simulink model "genset_imp_1"  (Simulink 7.6)
settings: Solver=ode23t  StartTime=0.0  StopTime=1  RelTol=1e-3
values from neighbouring files (symbols this model uses):
  AvrSat = 20*sqrt(2/3)    [articlerun.m]
  D_fw = 0.0    (= 0)    [articlerun.m]    (also in m1.m = 0.01)
  Davr = 0    [articlerun.m]
  Dgovernor = 10    [articlerun.m]
  droopAVR = 0.05    [articlerun.m]    (also in m1.m)
  droopGovernor = 0    [articlerun.m]    (also in m1.m)
  GovernorSamp = .01    (= 0.01)    [articlerun.m]
  H = 5.6    [articlerun.m]    (also in m1.m = 0.5*J_rotor*wbasem*wbasem/Sbase)
  Iavr = 0    [articlerun.m]
  Igovernor = 10    [articlerun.m]
  loadAmplitude = 0    [initArt.m]
  loadBias = 0.5    [initArt.m]
  loadfreq = 2*pi/loadT    (= 628.318530718)    [initArt.m]
  loadStep = 0    [initArt.m]
  loadStepTime = 15    [initArt.m]
  Pavr = 400    [articlerun.m]
  Pgovernor = 20    [articlerun.m]
  S_b = 325e6    (= 325000000)    [articlerun.m]    (also in m1.m)
  V_b = 26e3    (= 26000)    [articlerun.m]    (also in m1.m = 20000)
  w_b = 60*2*pi    (= 376.991118431)    [articlerun.m]    (also in m1.m)
undefined symbols (not defined in the file or in its folder): delayEngineRack, deltaomega, Genset, PMSlib, R_a, tau_e, Xbus
libraries: simulink x2
settings Model: Creator=tibnor  LastModifiedBy=tibnor  BufferReuse=off
settings OptimizationCC: OptimizeBlockIOStorage=off  BufferReuse=off  ExpressionFolding=off  LocalBlockOutputs=off

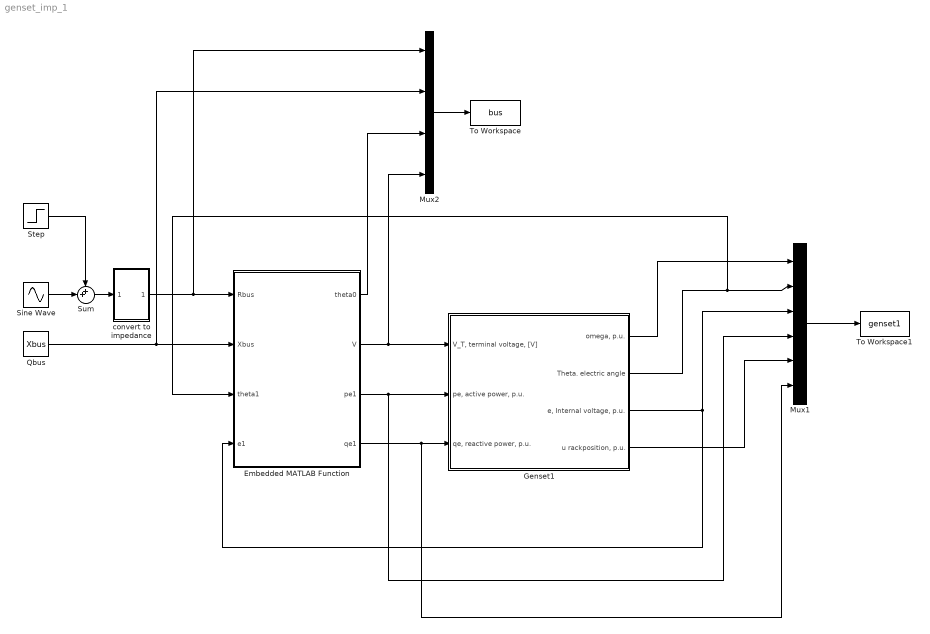
== system genset_imp_1 ==
  Embedded MATLAB Function : Stateflow chart  TreatAsAtomicUnit=on
  Genset1 : Subsystem  AncestorBlock=PMSlib/Genset
  Mux1 : Mux  Inputs=6
  Mux2 : Mux
  Qbus : Constant  Value=Xbus
  Sine Wave : Sin  Amplitude=loadAmplitude  Bias=loadBias  Frequency=loadfreq  SampleTime=0
  Step : Step  Time=loadStepTime  After=loadStep  SampleTime=0
  Sum : Sum  Inputs=++|
  To Workspace : ToWorkspace  VariableName=bus  SampleTime=-1  SaveFormat=Structure With Time
  To Workspace1 : ToWorkspace  VariableName=genset1  SampleTime=-1  SaveFormat=Structure With Time
  convert to impedance : Subsystem
  wires:
  Genset1/2(Theta. electric angle) -> Embedded MATLAB Function/3(theta1), Mux1/2
  Qbus/1 -> Embedded MATLAB Function/2(Xbus), Mux2/2
  Genset1/1("omega, p.u.") -> Mux1/1
  Mux2/1 -> To Workspace/1
  Embedded MATLAB Function/1(theta0) -> Mux2/3
  Mux1/1 -> To Workspace1/1
  Embedded MATLAB Function/4(qe1) -> Genset1/3("qe, reactive power, p.u."), Mux1/6
  Sine Wave/1 -> Sum/2
  Step/1 -> Sum/1
  Genset1/4("u rackposition, p.u.") -> Mux1/5
  Embedded MATLAB Function/3(pe1) -> Genset1/2("pe, active power, p.u."), Mux1/4
  Embedded MATLAB Function/2(V) -> Genset1/1("V_T, terminal voltage, [V]"), Mux2/4
  Genset1/3("e, Internal voltage, p.u.") -> Mux1/3, Embedded MATLAB Function/4(e1)
  Sum/1 -> convert to impedance/1(power)
  convert to impedance/1(resistance) -> Embedded MATLAB Function/1(Rbus), Mux2/1

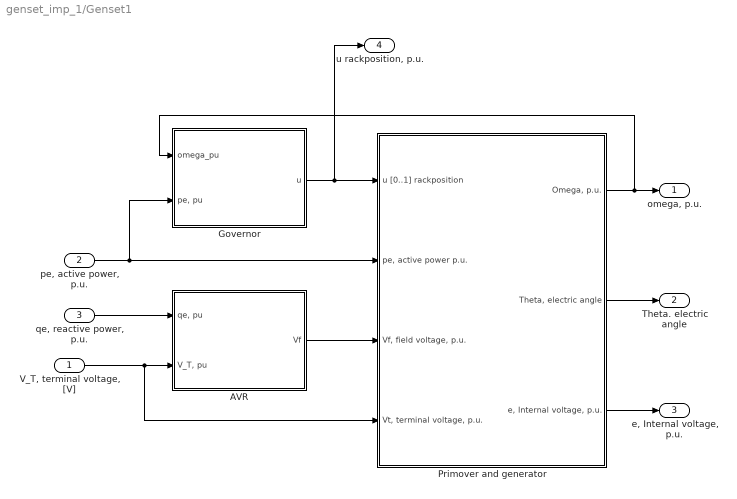
== system genset_imp_1/Genset1 ==
  "V_T, terminal voltage, [V]" : Inport
  "pe, active power, p.u." : Inport  Port=2
  "qe, reactive power, p.u." : Inport  Port=3
  AVR : Subsystem
  Governor : Subsystem
  Primover and generator : Subsystem
  "omega, p.u." : Outport
  Theta. electric angle : Outport  Port=2
  "e, Internal voltage, p.u." : Outport  Port=3
  "u rackposition, p.u." : Outport  Port=4
  wires:
  Primover and generator/2("Theta, electric angle") -> Theta. electric angle/1
  "pe, active power, p.u."/1 -> Governor/2("pe, pu"), Primover and generator/2("pe, active power p.u.")
  Primover and generator/3("e, Internal voltage, p.u.") -> "e, Internal voltage, p.u."/1
  Governor/1(u) -> Primover and generator/1(u [0..1] rackposition), "u rackposition, p.u."/1
  AVR/1(Vf) -> Primover and generator/3("Vf, field voltage, p.u.")
  "qe, reactive power, p.u."/1 -> AVR/1("qe, pu")
  "V_T, terminal voltage, [V]"/1 -> AVR/2("V_T, pu"), Primover and generator/4("Vt, terminal voltage, p.u.")
  Primover and generator/1("Omega, p.u.") -> "omega, p.u."/1, Governor/1(omega_pu)

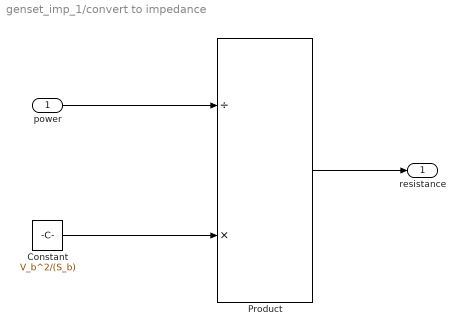
== system genset_imp_1/convert to impedance ==
  power : Inport
  Constant : Constant  Value=V_b^2/(S_b)
  Product : Product  Inputs=/*  RndMeth=Zero
  resistance : Outport
  wires:
  Constant/1 -> Product/2
  power/1 -> Product/1
  Product/1 -> resistance/1

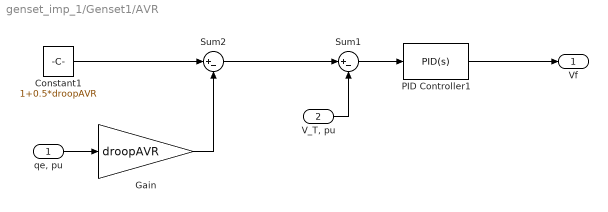
== system genset_imp_1/Genset1/AVR ==
  "qe, pu" : Inport
  "V_T, pu" : Inport  Port=2
  Constant1 : Constant  Value=1+0.5*droopAVR
  Gain : Gain  Gain=droopAVR
  PID Controller1 : simulink/Continuous/PID Controller  Controller=PID  TimeDomain=Continuous-time  SampleTime=1  IntegratorMethod=Forward Euler  FilterMethod=Forward Euler  Form=Parallel  P=Pavr  I=Iavr  D=Davr  N=100  InitialConditionSource=internal  InitialConditionForIntegrator=1  InitialConditionForFilter=0  ExternalReset=none  LimitOutput=on  UpperSaturationLimit=AvrSat  LowerSaturationLimit=-AvrSat  LinearizeAsGain=off  AntiWindupMode=none  Kb=1  TrackingMode=off  Kt=1  PParamMin=[]  PParamMax=[]  IParamMin=[]  IParamMax=[]  DParamMin=[]  DParamMax=[]  NParamMin=[]  NParamMax=[]  KbParamMin=[]  KbParamMax=[]  KtParamMin=[]  KtParamMax=[]  POutMin=[]  POutMax=[]  IOutMin=[]  IOutMax=[]  DOutMin=[]  DOutMax=[]  NOutMin=[]  NOutMax=[]  KbOutMin=[]  KbOutMax=[]  KtOutMin=[]  KtOutMax=[]  IntegratorOutMin=[]  IntegratorOutMax=[]  FilterOutMin=[]  FilterOutMax=[]  SumOutMin=[]  SumOutMax=[]  SumI1OutMin=[]  SumI1OutMax=[]  SumI2OutMin=[]  SumI2OutMax=[]  SumI3OutMin=[]  SumI3OutMax=[]  SumDOutMin=[]  SumDOutMax=[]  SaturationOutMin=[]  SaturationOutMax=[]  IntegratorContinuousStateAttributes=''  IntegratorStateMustResolveToSignalObject=off  IntegratorRTWStateStorageClass=Auto  FilterContinuousStateAttributes=''  FilterStateMustResolveToSignalObject=off  FilterRTWStateStorageClass=Auto
  Sum1 : Sum  Inputs=|+-
  Sum2 : Sum  Inputs=|+-
  Vf : Outport
  wires:
  Gain/1 -> Sum2/2
  "qe, pu"/1 -> Gain/1
  Sum2/1 -> Sum1/1
  Constant1/1 -> Sum2/1
  "V_T, pu"/1 -> Sum1/2
  PID Controller1/1 -> Vf/1
  Sum1/1 -> PID Controller1/1

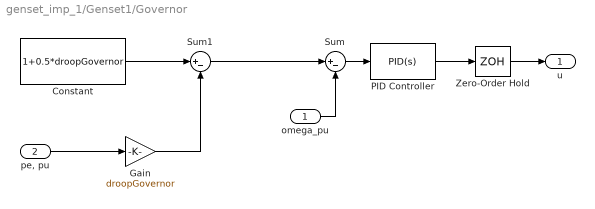
== system genset_imp_1/Genset1/Governor ==
  omega_pu : Inport
  "pe, pu" : Inport  Port=2
  Constant : Constant  Value=1+0.5*droopGovernor
  Gain : Gain  Gain=droopGovernor
  PID Controller : simulink/Continuous/PID Controller  Controller=PID  TimeDomain=Continuous-time  SampleTime=1  IntegratorMethod=Forward Euler  FilterMethod=Forward Euler  Form=Parallel  P=Pgovernor  I=Igovernor  D=Dgovernor  N=100  InitialConditionSource=internal  InitialConditionForIntegrator=0  InitialConditionForFilter=0  ExternalReset=none  LimitOutput=on  UpperSaturationLimit=2  LowerSaturationLimit=0  LinearizeAsGain=off  AntiWindupMode=none  Kb=1  TrackingMode=off  Kt=1  PParamMin=[]  PParamMax=[]  IParamMin=[]  IParamMax=[]  DParamMin=[]  DParamMax=[]  NParamMin=[]  NParamMax=[]  KbParamMin=[]  KbParamMax=[]  KtParamMin=[]  KtParamMax=[]  POutMin=[]  POutMax=[]  IOutMin=[]  IOutMax=[]  DOutMin=[]  DOutMax=[]  NOutMin=[]  NOutMax=[]  KbOutMin=[]  KbOutMax=[]  KtOutMin=[]  KtOutMax=[]  IntegratorOutMin=[]  IntegratorOutMax=[]  FilterOutMin=[]  FilterOutMax=[]  SumOutMin=[]  SumOutMax=[]  SumI1OutMin=[]  SumI1OutMax=[]  SumI2OutMin=[]  SumI2OutMax=[]  SumI3OutMin=[]  SumI3OutMax=[]  SumDOutMin=[]  SumDOutMax=[]  SaturationOutMin=[]  SaturationOutMax=[]  IntegratorContinuousStateAttributes=''  IntegratorStateMustResolveToSignalObject=off  IntegratorRTWStateStorageClass=Auto  FilterContinuousStateAttributes=''  FilterStateMustResolveToSignalObject=off  FilterRTWStateStorageClass=Auto
  Sum : Sum  Inputs=|+-
  Sum1 : Sum  Inputs=|+-
  Zero-Order Hold : ZeroOrderHold  SampleTime=GovernorSamp
  u : Outport
  wires:
  Gain/1 -> Sum1/2
  "pe, pu"/1 -> Gain/1
  Sum1/1 -> Sum/1
  Constant/1 -> Sum1/1
  omega_pu/1 -> Sum/2
  PID Controller/1 -> Zero-Order Hold/1
  Sum/1 -> PID Controller/1
  Zero-Order Hold/1 -> u/1

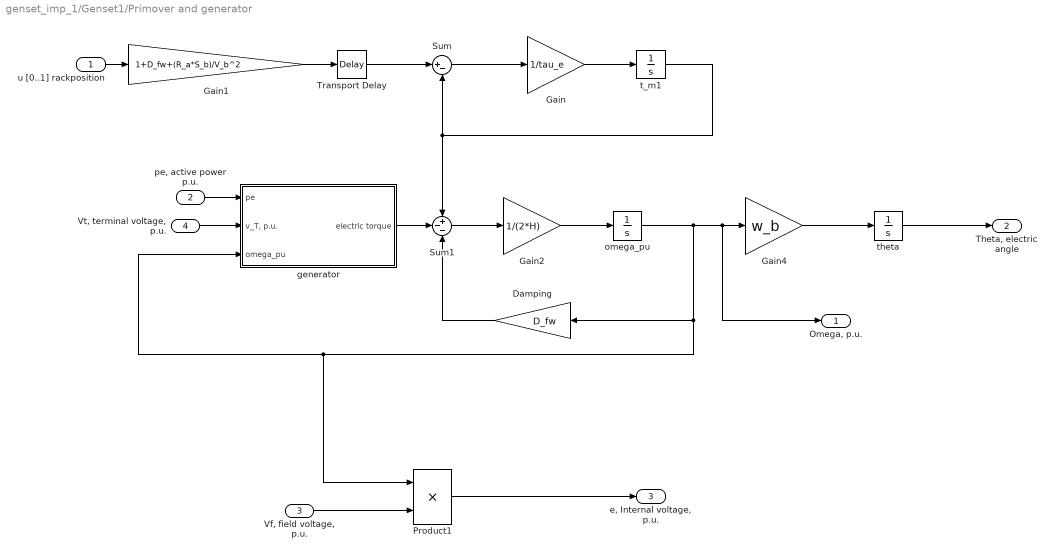
== system genset_imp_1/Genset1/Primover and generator ==
  u [0..1] rackposition : Inport
  "pe, active power p.u." : Inport  Port=2
  "Vf, field voltage, p.u." : Inport  Port=3
  "Vt, terminal voltage, p.u." : Inport  Port=4
  Damping : Gain  Gain=D_fw
  Gain : Gain  Gain=1/tau_e
  Gain1 : Gain  Gain=1+D_fw+(R_a*S_b)/V_b^2
  Gain2 : Gain  Gain=1/(2*H)
  Gain4 : Gain  Gain=w_b
  Product1 : Product  Inputs=**  RndMeth=Zero
  Sum : Sum  Inputs=|+-
  Sum1 : Sum  Inputs=+--
  Transport Delay : TransportDelay  DelayTime=delayEngineRack
  generator : Subsystem
  omega_pu : Integrator  InitialCondition=1
  t_m1 : Integrator
  theta : Integrator
  "Omega, p.u." : Outport
  "Theta, electric angle" : Outport  Port=2
  "e, Internal voltage, p.u." : Outport  Port=3
  wires:
  "pe, active power p.u."/1 -> generator/1(pe)
  "Vf, field voltage, p.u."/1 -> Product1/2
  Product1/1 -> "e, Internal voltage, p.u."/1
  u [0..1] rackposition/1 -> Gain1/1
  theta/1 -> "Theta, electric angle"/1
  Gain4/1 -> theta/1
  generator/1(electric torque) -> Sum1/2
  Damping/1 -> Sum1/3
  omega_pu/1 -> "Omega, p.u."/1, Gain4/1, generator/3(omega_pu), Product1/1, Damping/1
  Sum1/1 -> Gain2/1
  Gain2/1 -> omega_pu/1
  t_m1/1 -> Sum1/1, Sum/2
  Sum/1 -> Gain/1
  Gain1/1 -> Transport Delay/1
  Gain/1 -> t_m1/1
  "Vt, terminal voltage, p.u."/1 -> generator/2("v_T, p.u.")
  Transport Delay/1 -> Sum/1

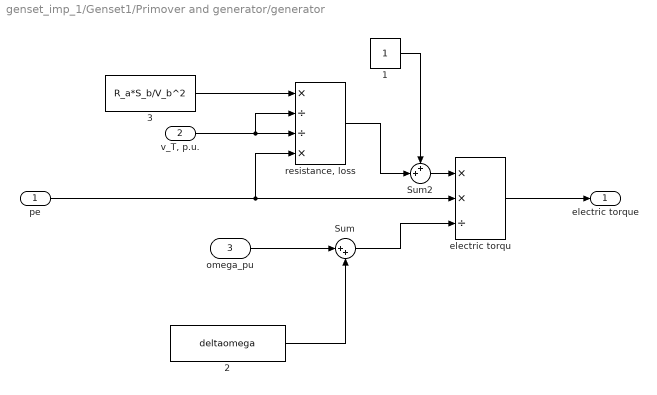
== system genset_imp_1/Genset1/Primover and generator/generator ==
  pe : Inport
  "v_T, p.u." : Inport  Port=2
  omega_pu : Inport  Port=3
  1 : Constant
  2 : Constant  Value=deltaomega
  3 : Constant  Value=R_a*S_b/V_b^2
  Sum : Sum  Inputs=|++
  Sum2 : Sum  Inputs=++|
  electric torqu : Product  Inputs=**/  RndMeth=Zero
  "resistance, loss" : Product  Inputs=*//*  RndMeth=Zero
  electric torque : Outport
  wires:
  2/1 -> Sum/2
  Sum/1 -> electric torqu/3
  omega_pu/1 -> Sum/1
  pe/1 -> electric torqu/2, "resistance, loss"/4
  electric torqu/1 -> electric torque/1
  Sum2/1 -> electric torqu/1
  "v_T, p.u."/1 -> "resistance, loss"/3, "resistance, loss"/2
  3/1 -> "resistance, loss"/1
  1/1 -> Sum2/1
  "resistance, loss"/1 -> Sum2/2

== matlab function Embedded MATLAB Function ==
  data: Rbus input double; Xbus input double; theta1 input double; e1 input double; theta0 output double; V output double; pe1 output double; qe1 output double
function [theta0,V,pe1,qe1] = fcn(Rbus,Xbus,theta1,e1)
Sb = 835e6;
Vb = 26e3;
ZLR = Rbus*Sb/Vb^2;
ZLX = 1j*Xbus*Sb/Vb^2;
ZL = 1/(1/ZLR+1/ZLX);
z1 = 0.003+1.8j;
e1 = e1*exp(1j*theta1);
VT = e1;
ZT = z1;
V0 = (ZL/(ZL+ZT))*VT;
S1 = V0*((e1-V0)/z1)';
pe1 = real(S1);
qe1 = imag(S1);
theta0 = angle(V0);
V = abs(V0);
